simulink model "model"  (R2014a)
(part 4 of 4)

  T_174586802__/RConn1 -- L_174586802/LConn1
  T_174586802__/RConn2 -- L_174586802/LConn2
  L_174586802/LConn3 -- T_174586802__/RConn3 -- bus230/LConn1
  T_172019051__/RConn1 -- L_172019051/LConn1
  T_172019051__/RConn2 -- L_172019051/LConn2
  L_172019051/LConn3 -- T_172019051__/RConn3 -- bus231/LConn1
  T_214649879__/RConn1 -- L_214649879/LConn1
  T_214649879__/RConn2 -- L_214649879/LConn2
  L_214649879/LConn3 -- T_214649879__/RConn3 -- bus232/LConn1
  T_171809316__/RConn1 -- L_171809316/LConn1
  T_171809316__/RConn2 -- L_171809316/LConn2
  L_171809316/LConn3 -- T_171809316__/RConn3 -- bus233/LConn1
  T_103275527__/RConn1 -- L_103275527/LConn1
  T_103275527__/RConn2 -- L_103275527/LConn2
  L_103275527/LConn3 -- T_103275527__/RConn3 -- bus234/LConn1
  T_103275559__/RConn1 -- L_103275559/LConn1
  T_103275559__/RConn2 -- L_103275559/LConn2
  L_103275559/LConn3 -- T_103275559__/RConn3 -- bus235/LConn1
  T_103275551__/RConn1 -- L_103275551/LConn1
  T_103275551__/RConn2 -- L_103275551/LConn2
  L_103275551/LConn3 -- T_103275551__/RConn3 -- bus236/LConn1
  T_209204254__/RConn1 -- L_209204254/LConn1
  T_209204254__/RConn2 -- L_209204254/LConn2
  L_209204254/LConn3 -- T_209204254__/RConn3 -- bus237/LConn1
  T_103560163__/RConn1 -- L_103560163/LConn1
  T_103560163__/RConn2 -- L_103560163/LConn2
  L_103560163/LConn3 -- T_103560163__/RConn3 -- bus238/LConn1
  T_124462106__/RConn1 -- L_124462106/LConn1
  T_124462106__/RConn2 -- L_124462106/LConn2
  L_124462106/LConn3 -- T_124462106__/RConn3 -- bus239/LConn1
  T_171630121__/RConn1 -- L_171630121/LConn1
  T_171630121__/RConn2 -- L_171630121/LConn2
  L_171630121/LConn3 -- T_171630121__/RConn3 -- bus240/LConn1
  T_142782984__/RConn1 -- L_142782984/LConn1
  T_142782984__/RConn2 -- L_142782984/LConn2
  L_142782984/LConn3 -- T_142782984__/RConn3 -- bus241/LConn1
  T_173582225__/RConn1 -- L_173582225/LConn1
  T_173582225__/RConn2 -- L_173582225/LConn2
  L_173582225/LConn3 -- T_173582225__/RConn3 -- bus242/LConn1
  T_153249112__/RConn1 -- L_153249112/LConn1
  T_153249112__/RConn2 -- L_153249112/LConn2
  L_153249112/LConn3 -- T_153249112__/RConn3 -- bus243/LConn1
  T_172590095__/RConn1 -- L_172590095/LConn1
  T_172590095__/RConn2 -- L_172590095/LConn2
  L_172590095/LConn3 -- T_172590095__/RConn3 -- bus244/LConn1
  T_172590108__/RConn1 -- L_172590108/LConn1
  T_172590108__/RConn2 -- L_172590108/LConn2
  L_172590108/LConn3 -- T_172590108__/RConn3 -- bus245/LConn1
  T_172590096__/RConn1 -- L_172590096/LConn1
  T_172590096__/RConn2 -- L_172590096/LConn2
  L_172590096/LConn3 -- T_172590096__/RConn3 -- bus246/LConn1
  T_172590097__/RConn1 -- L_172590097/LConn1
  T_172590097__/RConn2 -- L_172590097/LConn2
  L_172590097/LConn3 -- T_172590097__/RConn3 -- bus247/LConn1
  T_173612890__Garliavos_TP/RConn1 -- L_173612890/LConn1
  T_173612890__Garliavos_TP/RConn2 -- L_173612890/LConn2
  L_173612890/LConn3 -- T_173612890__Garliavos_TP/RConn3 -- bus248/LConn1
  T_218214432__/RConn1 -- L_218214432/LConn1
  T_218214432__/RConn2 -- L_218214432/LConn2
  L_218214432/LConn3 -- T_218214432__/RConn3 -- bus249/LConn1
  T_218216075_110000;35000;10000_/RConn1 -- L_218216075/LConn1
  T_218216075_110000;35000;10000_/RConn2 -- L_218216075/LConn2
  L_218216075/LConn3 -- T_218216075_110000;35000;10000_/RConn3 -- bus250/LConn1
  T_260552752_110000;35000;10000_/RConn1 -- L_260552752/LConn1
  T_260552752_110000;35000;10000_/RConn2 -- L_260552752/LConn2
  L_260552752/LConn3 -- T_260552752_110000;35000;10000_/RConn3 -- bus251/LConn1
  T_214455329__/RConn1 -- L_214455329/LConn1
  T_214455329__/RConn2 -- L_214455329/LConn2
  L_214455329/LConn3 -- T_214455329__/RConn3 -- bus252/LConn1
  T_210619011__/RConn1 -- L_210619011/LConn1
  T_210619011__/RConn2 -- L_210619011/LConn2
  L_210619011/LConn3 -- T_210619011__/RConn3 -- bus253/LConn1
  T_280078882__/RConn1 -- L_280078882/LConn1
  T_280078882__/RConn2 -- L_280078882/LConn2
  L_280078882/LConn3 -- T_280078882__/RConn3 -- bus254/LConn1
  T_221105370__/RConn1 -- L_221105370/LConn1
  T_221105370__/RConn2 -- L_221105370/LConn2
  L_221105370/LConn3 -- T_221105370__/RConn3 -- bus255/LConn1
  T_151237667__/RConn1 -- L_151237667/LConn1
  T_151237667__/RConn2 -- L_151237667/LConn2
  L_151237667/LConn3 -- T_151237667__/RConn3 -- bus256/LConn1
  T_134987741__/RConn1 -- L_134987741/LConn1
  T_134987741__/RConn2 -- L_134987741/LConn2
  L_134987741/LConn3 -- T_134987741__/RConn3 -- bus257/LConn1
  T_103275575__/RConn1 -- L_103275575/LConn1
  T_103275575__/RConn2 -- L_103275575/LConn2
  L_103275575/LConn3 -- T_103275575__/RConn3 -- bus258/LConn1
  T_150992936_110000;35000;fixme_/RConn1 -- L_150992936/LConn1
  T_150992936_110000;35000;fixme_/RConn2 -- L_150992936/LConn2
  L_150992936/LConn3 -- T_150992936_110000;35000;fixme_/RConn3 -- bus259/LConn1
  T_151783148_110000;fixme_/RConn1 -- L_151783148/LConn1
  T_151783148_110000;fixme_/RConn2 -- L_151783148/LConn2
  L_151783148/LConn3 -- T_151783148_110000;fixme_/RConn3 -- bus260/LConn1
  T_103554499__/RConn1 -- L_103554499/LConn1
  T_103554499__/RConn2 -- L_103554499/LConn2
  L_103554499/LConn3 -- T_103554499__/RConn3 -- bus261/LConn1
  T_207755730__/RConn1 -- L_207755730/LConn1
  T_207755730__/RConn2 -- L_207755730/LConn2
  L_207755730/LConn3 -- T_207755730__/RConn3 -- bus262/LConn1
  T_207755729__/RConn1 -- L_207755729/LConn1
  T_207755729__/RConn2 -- L_207755729/LConn2
  L_207755729/LConn3 -- T_207755729__/RConn3 -- bus263/LConn1
  T_218047622__/RConn1 -- L_218047622/LConn1
  T_218047622__/RConn2 -- L_218047622/LConn2
  L_218047622/LConn3 -- T_218047622__/RConn3 -- bus264/LConn1
  T_218223016__/RConn1 -- L_218223016/LConn1
  T_218223016__/RConn2 -- L_218223016/LConn2
  L_218223016/LConn3 -- T_218223016__/RConn3 -- bus265/LConn1
  T_151783156__/RConn1 -- L_151783156/LConn1
  T_151783156__/RConn2 -- L_151783156/LConn2
  L_151783156/LConn3 -- T_151783156__/RConn3 -- bus266/LConn1
  T_172407405__/RConn1 -- L_172407405/LConn1
  T_172407405__/RConn2 -- L_172407405/LConn2
  L_172407405/LConn3 -- T_172407405__/RConn3 -- bus267/LConn1
  T_218223015__/RConn1 -- L_218223015/LConn1
  T_218223015__/RConn2 -- L_218223015/LConn2
  L_218223015/LConn3 -- T_218223015__/RConn3 -- bus268/LConn1
  T_171406899__/RConn1 -- L_171406899/LConn1
  T_171406899__/RConn2 -- L_171406899/LConn2
  L_171406899/LConn3 -- T_171406899__/RConn3 -- bus269/LConn1
  T_175315244__/RConn1 -- L_175315244/LConn1
  T_175315244__/RConn2 -- L_175315244/LConn2
  L_175315244/LConn3 -- T_175315244__/RConn3 -- bus270/LConn1
  T_172978107__/RConn1 -- L_172978107/LConn1
  T_172978107__/RConn2 -- L_172978107/LConn2
  L_172978107/LConn3 -- T_172978107__/RConn3 -- bus271/LConn1
  T_210619008__/RConn1 -- L_210619008/LConn1
  T_210619008__/RConn2 -- L_210619008/LConn2
  L_210619008/LConn3 -- T_210619008__/RConn3 -- bus272/LConn1
  T_257507721__/RConn1 -- L_257507721/LConn1
  T_257507721__/RConn2 -- L_257507721/LConn2
  L_257507721/LConn3 -- T_257507721__/RConn3 -- bus273/LConn1
  T_210612962__/RConn1 -- L_210612962/LConn1
  T_210612962__/RConn2 -- L_210612962/LConn2
  L_210612962/LConn3 -- T_210612962__/RConn3 -- bus274/LConn1
  T_210609525__/RConn1 -- L_210609525/LConn1
  T_210609525__/RConn2 -- L_210609525/LConn2
  L_210609525/LConn3 -- T_210609525__/RConn3 -- bus275/LConn1
  T_104774544__/RConn1 -- L_104774544/LConn1
  T_104774544__/RConn2 -- L_104774544/LConn2
  L_104774544/LConn3 -- T_104774544__/RConn3 -- bus276/LConn1
  T_173944057__/RConn1 -- L_173944057/LConn1
  T_173944057__/RConn2 -- L_173944057/LConn2
  L_173944057/LConn3 -- T_173944057__/RConn3 -- bus277/LConn1
  T_173944061__/RConn1 -- L_173944061/LConn1
  T_173944061__/RConn2 -- L_173944061/LConn2
  L_173944061/LConn3 -- T_173944061__/RConn3 -- bus278/LConn1
  T_171630144__/RConn1 -- L_171630144/LConn1
  T_171630144__/RConn2 -- L_171630144/LConn2
  L_171630144/LConn3 -- T_171630144__/RConn3 -- bus279/LConn1
  T_171630156__/RConn1 -- L_171630156/LConn1
  T_171630156__/RConn2 -- L_171630156/LConn2
  L_171630156/LConn3 -- T_171630156__/RConn3 -- bus280/LConn1
  T_171630149__/RConn1 -- L_171630149/LConn1
  T_171630149__/RConn2 -- L_171630149/LConn2
  L_171630149/LConn3 -- T_171630149__/RConn3 -- bus281/LConn1
  T_171630143__/RConn1 -- L_171630143/LConn1
  T_171630143__/RConn2 -- L_171630143/LConn2
  L_171630143/LConn3 -- T_171630143__/RConn3 -- bus282/LConn1
  T_192672898__/RConn1 -- L_192672898/LConn1
  T_192672898__/RConn2 -- L_192672898/LConn2
  L_192672898/LConn3 -- T_192672898__/RConn3 -- bus283/LConn1
  T_192646598__/RConn1 -- L_192646598/LConn1
  T_192646598__/RConn2 -- L_192646598/LConn2
  L_192646598/LConn3 -- T_192646598__/RConn3 -- bus284/LConn1
  T_171630157__/RConn1 -- L_171630157/LConn1
  T_171630157__/RConn2 -- L_171630157/LConn2
  L_171630157/LConn3 -- T_171630157__/RConn3 -- bus285/LConn1
  T_105587267__/RConn1 -- L_105587267/LConn1
  T_105587267__/RConn2 -- L_105587267/LConn2
  L_105587267/LConn3 -- T_105587267__/RConn3 -- bus286/LConn1
  T_243085462__/RConn1 -- L_243085462/LConn1
  T_243085462__/RConn2 -- L_243085462/LConn2
  L_243085462/LConn3 -- T_243085462__/RConn3 -- bus287/LConn1
  T_171630153_110000;fixme_/RConn1 -- L_171630153/LConn1
  T_171630153_110000;fixme_/RConn2 -- L_171630153/LConn2
  L_171630153/LConn3 -- T_171630153_110000;fixme_/RConn3 -- bus288/LConn1
  T_104774536__/RConn1 -- L_104774536/LConn1
  T_104774536__/RConn2 -- L_104774536/LConn2
  L_104774536/LConn3 -- T_104774536__/RConn3 -- bus289/LConn1
  T_239589747_110000;fixme_/RConn1 -- L_239589747/LConn1
  T_239589747_110000;fixme_/RConn2 -- L_239589747/LConn2
  L_239589747/LConn3 -- T_239589747_110000;fixme_/RConn3 -- bus290/LConn1
  T_172019117__/RConn1 -- L_172019117/LConn1
  T_172019117__/RConn2 -- L_172019117/LConn2
  L_172019117/LConn3 -- T_172019117__/RConn3 -- bus291/LConn1
  T_172019087__/RConn1 -- L_172019087/LConn1
  T_172019087__/RConn2 -- L_172019087/LConn2
  L_172019087/LConn3 -- T_172019087__/RConn3 -- bus292/LConn1
  T_192764347_110000;fixme_/RConn1 -- L_192764347/LConn1
  T_192764347_110000;fixme_/RConn2 -- L_192764347/LConn2
  L_192764347/LConn3 -- T_192764347_110000;fixme_/RConn3 -- bus293/LConn1
  T_192764331__/RConn1 -- L_192764331/LConn1
  T_192764331__/RConn2 -- L_192764331/LConn2
  L_192764331/LConn3 -- T_192764331__/RConn3 -- bus294/LConn1
  T_192764337_110000;fixme_/RConn1 -- L_192764337/LConn1
  T_192764337_110000;fixme_/RConn2 -- L_192764337/LConn2
  L_192764337/LConn3 -- T_192764337_110000;fixme_/RConn3 -- bus295/LConn1
  T_210557029_110000;35000;fixme_/RConn1 -- L_210557029/LConn1
  T_210557029_110000;35000;fixme_/RConn2 -- L_210557029/LConn2
  L_210557029/LConn3 -- T_210557029_110000;35000;fixme_/RConn3 -- bus296/LConn1
  T_181769867__/RConn1 -- L_181769867/LConn1
  T_181769867__/RConn2 -- L_181769867/LConn2
  L_181769867/LConn3 -- T_181769867__/RConn3 -- bus297/LConn1
  T_173582216__/RConn1 -- L_173582216/LConn1
  T_173582216__/RConn2 -- L_173582216/LConn2
  L_173582216/LConn3 -- T_173582216__/RConn3 -- bus298/LConn1
  T_231990061__/RConn1 -- L_231990061/LConn1
  T_231990061__/RConn2 -- L_231990061/LConn2
  L_231990061/LConn3 -- T_231990061__/RConn3 -- bus299/LConn1
  T_192672875__/RConn1 -- L_192672875/LConn1
  T_192672875__/RConn2 -- L_192672875/LConn2
  L_192672875/LConn3 -- T_192672875__/RConn3 -- bus300/LConn1
  T_192677018__/RConn1 -- L_192677018/LConn1
  T_192677018__/RConn2 -- L_192677018/LConn2
  L_192677018/LConn3 -- T_192677018__/RConn3 -- bus301/LConn1
  T_192672905__/RConn1 -- L_192672905/LConn1
  T_192672905__/RConn2 -- L_192672905/LConn2
  L_192672905/LConn3 -- T_192672905__/RConn3 -- bus302/LConn1
  T_192672914__/RConn1 -- L_192672914/LConn1
  T_192672914__/RConn2 -- L_192672914/LConn2
  L_192672914/LConn3 -- T_192672914__/RConn3 -- bus303/LConn1
  T_172178550__/RConn1 -- L_172178550/LConn1
  T_172178550__/RConn2 -- L_172178550/LConn2
  L_172178550/LConn3 -- T_172178550__/RConn3 -- bus304/LConn1
  T_172178562__/RConn1 -- L_172178562/LConn1
  T_172178562__/RConn2 -- L_172178562/LConn2
  L_172178562/LConn3 -- T_172178562__/RConn3 -- bus305/LConn1
  T_172178551__/RConn1 -- L_172178551/LConn1
  T_172178551__/RConn2 -- L_172178551/LConn2
  L_172178551/LConn3 -- T_172178551__/RConn3 -- bus306/LConn1
  T_172178560__/RConn1 -- L_172178560/LConn1
  T_172178560__/RConn2 -- L_172178560/LConn2
  L_172178560/LConn3 -- T_172178560__/RConn3 -- bus307/LConn1
  T_172178563__/RConn1 -- L_172178563/LConn1
  T_172178563__/RConn2 -- L_172178563/LConn2
  L_172178563/LConn3 -- T_172178563__/RConn3 -- bus308/LConn1
  T_226292390__/RConn1 -- L_226292390/LConn1
  T_226292390__/RConn2 -- L_226292390/LConn2
  L_226292390/LConn3 -- T_226292390__/RConn3 -- bus309/LConn1
  T_172394924__/RConn1 -- L_172394924/LConn1
  T_172394924__/RConn2 -- L_172394924/LConn2
  L_172394924/LConn3 -- T_172394924__/RConn3 -- bus310/LConn1
  T_172394893__/RConn1 -- L_172394893/LConn1
  T_172394893__/RConn2 -- L_172394893/LConn2
  L_172394893/LConn3 -- T_172394893__/RConn3 -- bus311/LConn1
  T_220986987__/RConn1 -- L_220986987/LConn1
  T_220986987__/RConn2 -- L_220986987/LConn2
  L_220986987/LConn3 -- T_220986987__/RConn3 -- bus312/LConn1
  T_173582226__/RConn1 -- L_173582226/LConn1
  T_173582226__/RConn2 -- L_173582226/LConn2
  L_173582226/LConn3 -- T_173582226__/RConn3 -- bus313/LConn1
  T_220989437__/RConn1 -- L_220989437/LConn1
  T_220989437__/RConn2 -- L_220989437/LConn2
  L_220989437/LConn3 -- T_220989437__/RConn3 -- bus314/LConn1
  T_127212679__Noreikiškių_TP/RConn1 -- L_127212679/LConn1
  T_127212679__Noreikiškių_TP/RConn2 -- L_127212679/LConn2
  L_127212679/LConn3 -- T_127212679__Noreikiškių_TP/RConn3 -- bus315/LConn1
  T_130577811__Vilijampolės_TP/RConn1 -- L_130577811/LConn1
  T_130577811__Vilijampolės_TP/RConn2 -- L_130577811/LConn2
  L_130577811/LConn3 -- T_130577811__Vilijampolės_TP/RConn3 -- bus316/LConn1
  T_172019115__Aleksoto_TP/RConn1 -- L_172019115/LConn1
  T_172019115__Aleksoto_TP/RConn2 -- L_172019115/LConn2
  L_172019115/LConn3 -- T_172019115__Aleksoto_TP/RConn3 -- bus317/LConn1
  T_210555392_110000;35000;fixme_/RConn1 -- L_210555392/LConn1
  T_210555392_110000;35000;fixme_/RConn2 -- L_210555392/LConn2
  L_210555392/LConn3 -- T_210555392_110000;35000;fixme_/RConn3 -- bus318/LConn1
  T_210551439__/RConn1 -- L_210551439/LConn1
  T_210551439__/RConn2 -- L_210551439/LConn2
  L_210551439/LConn3 -- T_210551439__/RConn3 -- bus319/LConn1
  T_210550993__/RConn1 -- L_210550993/LConn1
  T_210550993__/RConn2 -- L_210550993/LConn2
  L_210550993/LConn3 -- T_210550993__/RConn3 -- bus320/LConn1
  T_88726161__Eigulių_TP/RConn1 -- L_88726161/LConn1
  T_88726161__Eigulių_TP/RConn2 -- L_88726161/LConn2
  L_88726161/LConn3 -- T_88726161__Eigulių_TP/RConn3 -- bus321/LConn1
  T_130577812__Šilainių_TP/RConn1 -- L_130577812/LConn1
  T_130577812__Šilainių_TP/RConn2 -- L_130577812/LConn2
  L_130577812/LConn3 -- T_130577812__Šilainių_TP/RConn3 -- bus322/LConn1
  T_173593029__Šilko_TP/RConn1 -- L_173593029/LConn1
  T_173593029__Šilko_TP/RConn2 -- L_173593029/LConn2
  L_173593029/LConn3 -- T_173593029__Šilko_TP/RConn3 -- bus323/LConn1
  T_192764327__/RConn1 -- L_192764327/LConn1
  T_192764327__/RConn2 -- L_192764327/LConn2
  L_192764327/LConn3 -- T_192764327__/RConn3 -- bus324/LConn1
  T_210449206__/RConn1 -- L_210449206/LConn1
  T_210449206__/RConn2 -- L_210449206/LConn2
  L_210449206/LConn3 -- T_210449206__/RConn3 -- bus325/LConn1
  T_171868832__/RConn1 -- L_171868832/LConn1
  T_171868832__/RConn2 -- L_171868832/LConn2
  L_171868832/LConn3 -- T_171868832__/RConn3 -- bus326/LConn1
  T_220065702__/RConn1 -- L_220065702/LConn1
  T_220065702__/RConn2 -- L_220065702/LConn2
  L_220065702/LConn3 -- T_220065702__/RConn3 -- bus327/LConn1
  T_220915873__/RConn1 -- L_220915873/LConn1
  T_220915873__/RConn2 -- L_220915873/LConn2
  L_220915873/LConn3 -- T_220915873__/RConn3 -- bus328/LConn1
  T_173591498__/RConn1 -- L_173591498/LConn1
  T_173591498__/RConn2 -- L_173591498/LConn2
  L_173591498/LConn3 -- T_173591498__/RConn3 -- bus329/LConn1
  T_173944056__/RConn1 -- L_173944056/LConn1
  T_173944056__/RConn2 -- L_173944056/LConn2
  L_173944056/LConn3 -- T_173944056__/RConn3 -- bus330/LConn1
  T_173591502__/RConn1 -- L_173591502/LConn1
  T_173591502__/RConn2 -- L_173591502/LConn2
  L_173591502/LConn3 -- T_173591502__/RConn3 -- bus331/LConn1
  T_173591500__/RConn1 -- L_173591500/LConn1
  T_173591500__/RConn2 -- L_173591500/LConn2
  L_173591500/LConn3 -- T_173591500__/RConn3 -- bus332/LConn1
  T_215632387__/RConn1 -- L_215632387/LConn1
  T_215632387__/RConn2 -- L_215632387/LConn2
  L_215632387/LConn3 -- T_215632387__/RConn3 -- bus333/LConn1
  T_171229484__/RConn1 -- L_171229484/LConn1
  T_171229484__/RConn2 -- L_171229484/LConn2
  L_171229484/LConn3 -- T_171229484__/RConn3 -- bus334/LConn1
  T_75909941__Bubių_pastotė/RConn1 -- L_75909941/LConn1
  T_75909941__Bubių_pastotė/RConn2 -- L_75909941/LConn2
  L_75909941/LConn3 -- T_75909941__Bubių_pastotė/RConn3 -- bus335/LConn1
  T_99049777__Gubernijos_pastotė/RConn1 -- L_99049777/LConn1
  T_99049777__Gubernijos_pastotė/RConn2 -- L_99049777/LConn2
  L_99049777/LConn3 -- T_99049777__Gubernijos_pastotė/RConn3 -- bus336/LConn1
  T_296374470__/RConn1 -- L_296374470/LConn1
  T_296374470__/RConn2 -- L_296374470/LConn2
  L_296374470/LConn3 -- T_296374470__/RConn3 -- bus337/LConn1
  T_187242275__/RConn1 -- L_187242275/LConn1
  T_187242275__/RConn2 -- L_187242275/LConn2
  L_187242275/LConn3 -- T_187242275__/RConn3 -- bus338/LConn1
  T_174045384__/RConn1 -- L_174045384/LConn1
  T_174045384__/RConn2 -- L_174045384/LConn2
  L_174045384/LConn3 -- T_174045384__/RConn3 -- bus339/LConn1
  T_171406897__/RConn1 -- L_171406897/LConn1
  T_171406897__/RConn2 -- L_171406897/LConn2
  L_171406897/LConn3 -- T_171406897__/RConn3 -- bus340/LConn1
  T_219084048__/RConn1 -- L_219084048/LConn1
  T_219084048__/RConn2 -- L_219084048/LConn2
  L_219084048/LConn3 -- T_219084048__/RConn3 -- bus341/LConn1
  T_192764330__/RConn1 -- L_192764330/LConn1
  T_192764330__/RConn2 -- L_192764330/LConn2
  L_192764330/LConn3 -- T_192764330__/RConn3 -- bus342/LConn1
  T_219077432_110000;fixme_/RConn1 -- L_219077432/LConn1
  T_219077432_110000;fixme_/RConn2 -- L_219077432/LConn2
  L_219077432/LConn3 -- T_219077432_110000;fixme_/RConn3 -- bus343/LConn1
  T_149815795_110000;35000;fixme_/RConn1 -- L_149815795/LConn1
  T_149815795_110000;35000;fixme_/RConn2 -- L_149815795/LConn2
  L_149815795/LConn3 -- T_149815795_110000;35000;fixme_/RConn3 -- bus344/LConn1
  T_149408618__/RConn1 -- L_149408618/LConn1
  T_149408618__/RConn2 -- L_149408618/LConn2
  L_149408618/LConn3 -- T_149408618__/RConn3 -- bus345/LConn1
  T_95066982__/RConn1 -- L_95066982/LConn1
  T_95066982__/RConn2 -- L_95066982/LConn2
  L_95066982/LConn3 -- T_95066982__/RConn3 -- bus346/LConn1
  T_95866738__/RConn1 -- L_95866738/LConn1
  T_95866738__/RConn2 -- L_95866738/LConn2
  L_95866738/LConn3 -- T_95866738__/RConn3 -- bus347/LConn1
  T_217323242__/RConn1 -- L_217323242/LConn1
  T_217323242__/RConn2 -- L_217323242/LConn2
  L_217323242/LConn3 -- T_217323242__/RConn3 -- bus348/LConn1
  T_192672903__/RConn1 -- L_192672903/LConn1
  T_192672903__/RConn2 -- L_192672903/LConn2
  L_192672903/LConn3 -- T_192672903__/RConn3 -- bus349/LConn1
  T_173944045__/RConn1 -- L_173944045/LConn1
  T_173944045__/RConn2 -- L_173944045/LConn2
  L_173944045/LConn3 -- T_173944045__/RConn3 -- bus350/LConn1
  T_173944055__/RConn1 -- L_173944055/LConn1
  T_173944055__/RConn2 -- L_173944055/LConn2
  L_173944055/LConn3 -- T_173944055__/RConn3 -- bus351/LConn1
  T_173944047__/RConn1 -- L_173944047/LConn1
  T_173944047__/RConn2 -- L_173944047/LConn2
  L_173944047/LConn3 -- T_173944047__/RConn3 -- bus352/LConn1
  T_192702885__/RConn1 -- L_192702885/LConn1
  T_192702885__/RConn2 -- L_192702885/LConn2
  L_192702885/LConn3 -- T_192702885__/RConn3 -- bus353/LConn1
  T_280269221__/RConn1 -- L_280269221/LConn1
  T_280269221__/RConn2 -- L_280269221/LConn2
  L_280269221/LConn3 -- T_280269221__/RConn3 -- bus354/LConn1
  T_106172865__/RConn1 -- L_106172865/LConn1
  T_106172865__/RConn2 -- L_106172865/LConn2
  L_106172865/LConn3 -- T_106172865__/RConn3 -- bus355/LConn1
  T_176323123__/RConn1 -- L_176323123/LConn1
  T_176323123__/RConn2 -- L_176323123/LConn2
  L_176323123/LConn3 -- T_176323123__/RConn3 -- bus356/LConn1
  T_99049787__Zoknių_pastotė/RConn1 -- L_99049787/LConn1
  T_99049787__Zoknių_pastotė/RConn2 -- L_99049787/LConn2
  L_99049787/LConn3 -- T_99049787__Zoknių_pastotė/RConn3 -- bus357/LConn1
  T_172018985__/RConn1 -- L_172018985/LConn1
  T_172018985__/RConn2 -- L_172018985/LConn2
  L_172018985/LConn3 -- T_172018985__/RConn3 -- bus358/LConn1
  T_95066966__Rėkyvos_pastotė/RConn1 -- L_95066966/LConn1
  T_95066966__Rėkyvos_pastotė/RConn2 -- L_95066966/LConn2
  L_95066966/LConn3 -- T_95066966__Rėkyvos_pastotė/RConn3 -- bus359/LConn1
  T_210457043__/RConn1 -- L_210457043/LConn1
  T_210457043__/RConn2 -- L_210457043/LConn2
  L_210457043/LConn3 -- T_210457043__/RConn3 -- bus360/LConn1
  T_210457037_330000;110000;10000_/RConn1 -- L_210457037/LConn1
  T_210457037_330000;110000;10000_/RConn2 -- L_210457037/LConn2
  L_210457037/LConn3 -- T_210457037_330000;110000;10000_/RConn3 -- bus361/LConn1
  T_99049810_110000;35000;fixme_/RConn1 -- L_99049810/LConn1
  T_99049810_110000;35000;fixme_/RConn2 -- L_99049810/LConn2
  L_99049810/LConn3 -- T_99049810_110000;35000;fixme_/RConn3 -- bus362/LConn1
  T_192764316__/RConn1 -- L_192764316/LConn1
  T_192764316__/RConn2 -- L_192764316/LConn2
  L_192764316/LConn3 -- T_192764316__/RConn3 -- bus363/LConn1
  T_192764310__/RConn1 -- L_192764310/LConn1
  T_192764310__/RConn2 -- L_192764310/LConn2
  L_192764310/LConn3 -- T_192764310__/RConn3 -- bus364/LConn1
  T_135644003__/RConn1 -- L_135644003/LConn1
  T_135644003__/RConn2 -- L_135644003/LConn2
  L_135644003/LConn3 -- T_135644003__/RConn3 -- bus365/LConn1
  T_257684865__/RConn1 -- L_257684865/LConn1
  T_257684865__/RConn2 -- L_257684865/LConn2
  L_257684865/LConn3 -- T_257684865__/RConn3 -- bus366/LConn1
  T_257684864__/RConn1 -- L_257684864/LConn1
  T_257684864__/RConn2 -- L_257684864/LConn2
  L_257684864/LConn3 -- T_257684864__/RConn3 -- bus367/LConn1
  T_173582215__/RConn1 -- L_173582215/LConn1
  T_173582215__/RConn2 -- L_173582215/LConn2
  L_173582215/LConn3 -- T_173582215__/RConn3 -- bus368/LConn1
  T_217391080__/RConn1 -- L_217391080/LConn1
  T_217391080__/RConn2 -- L_217391080/LConn2
  L_217391080/LConn3 -- T_217391080__/RConn3 -- bus369/LConn1
  T_151097769__/RConn1 -- L_151097769/LConn1
  T_151097769__/RConn2 -- L_151097769/LConn2
  L_151097769/LConn3 -- T_151097769__/RConn3 -- bus370/LConn1
  T_172445102__/RConn1 -- L_172445102/LConn1
  T_172445102__/RConn2 -- L_172445102/LConn2
  L_172445102/LConn3 -- T_172445102__/RConn3 -- bus371/LConn1
  T_172590050_330000_/RConn1 -- L_172590050/LConn1
  T_172590050_330000_/RConn2 -- L_172590050/LConn2
  L_172590050/LConn3 -- T_172590050_330000_/RConn3 -- bus372/LConn1
  T_29428018_330000_ПС_330_кВ_Гродно/RConn1 -- L_29428018/LConn1
  T_29428018_330000_ПС_330_кВ_Гродно/RConn2 -- L_29428018/LConn2
  L_29428018/LConn3 -- T_29428018_330000_ПС_330_кВ_Гродно/RConn3 -- bus373/LConn1
  T_268781050_330000_Bitėnai_Elektros_Tiltas/RConn1 -- L_268781050/LConn1
  T_268781050_330000_Bitėnai_Elektros_Tiltas/RConn2 -- L_268781050/LConn2
  L_268781050/LConn3 -- T_268781050_330000_Bitėnai_Elektros_Tiltas/RConn3 -- bus374/LConn1
  T_197911127_330000;110000;15000;6000_ПС_330_кВ_«Советск»/RConn1 -- L_197911127/LConn1
  T_197911127_330000;110000;15000;6000_ПС_330_кВ_«Советск»/RConn2 -- L_197911127/LConn2
  L_197911127/LConn3 -- T_197911127_330000;110000;15000;6000_ПС_330_кВ_«Советск»/RConn3 -- bus375/LConn1
  T_220065689__/RConn1 -- L_220065689/LConn1
  T_220065689__/RConn2 -- L_220065689/LConn2
  L_220065689/LConn3 -- T_220065689__/RConn3 -- bus376/LConn1
